simulink library "trans_resistance"  (R2020b)
settings: Solver=VariableStepAuto  StartTime=0.0  StopTime=10.0  RelTol=1e-3
values from neighbouring files (symbols this model uses):
  m = 2000    [Projektskript.m]    (also in init.m)
settings Model: Creator=janbantle  LastModifiedBy=Johnathy

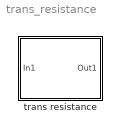
== system trans_resistance ==
  trans resistance : Subsystem

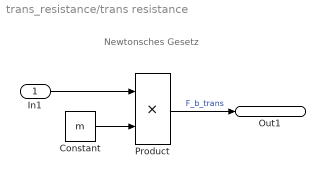
== system trans_resistance/trans resistance ==
  note: Newtonsches Gesetz
  In1 : Inport
  Constant : Constant  Value=m
  Product : Product
  Out1 : Outport
  wires:
  Product/1 -> Out1/1  "F_b_trans"
  Constant/1 -> Product/2
  In1/1 -> Product/1
